simulink model "sim_velo_control_PD_a_b_cCompensate"  (R2020b)
settings: Solver=FixedStepAuto  StartTime=0.0  StopTime=120  FixedStep=0.01  RelTol=1e-3
libraries: pid_lib x1
settings Model: Creator=User  LastModifiedBy=tuna
settings ConfigComp: PLC_TargetIDE=codesys23

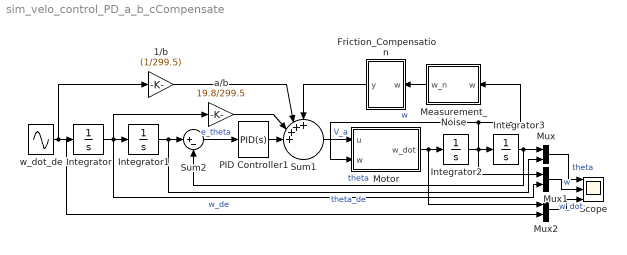
== system sim_velo_control_PD_a_b_cCompensate ==
  1/b : Gain  Gain=(1/299.5)
  Friction_Compensation : MATLAB Function  TreatAsAtomicUnit=on
  Integrator : Integrator  InitialCondition=15
  Integrator1 : Integrator
  Integrator2 : Integrator
  Integrator3 : Integrator
  Measurement_Noise : MATLAB Function  TreatAsAtomicUnit=on
  Motor : MATLAB Function  TreatAsAtomicUnit=on
  Mux : Mux  Inputs=2
  Mux1 : Mux  Inputs=2
  Mux2 : Mux  Inputs=2
  PID Controller1 : pid_lib/PID Controller  Controller=PID  Form=Parallel  TimeDomain=Continuous-time  UseExternalTs=off  SampleTime=-1  IntegratorMethod=Forward Euler  FilterMethod=Forward Euler  ControllerParametersSource=internal  P=3.8093  I=0  D=0.1596  UseFilter=on  N=100  TunerSelectOption=Transfer Function Based (PID Tuner App)  InitialConditionSource=internal  InitialConditionForIntegrator=0  InitialConditionForFilter=0  DifferentiatorICPrevScaledInput=0  ExternalReset=none  TrackingMode=off  Kt=1  LimitOutput=off  SatLimitsSource=internal  UpperSaturationLimit=inf  LowerSaturationLimit=-inf  LinearizeAsGain=on  AntiWindupMode=none  Kb=1  POutMin=[]  POutMax=[]  IOutMin=[]  IOutMax=[]  DOutMin=[]  DOutMax=[]  NOutMin=[]  NOutMax=[]  SumOutMin=[]  SumOutMax=[]  SaturationOutMin=[]  SaturationOutMax=[]  PParamMin=[]  PParamMax=[]  IParamMin=[]  IParamMax=[]  DParamMin=[]  DParamMax=[]  NParamMin=[]  NParamMax=[]  KbParamMin=[]  KbParamMax=[]  KtParamMin=[]  KtParamMax=[]  KbOutMin=[]  KbOutMax=[]  KtOutMin=[]  KtOutMax=[]  IntegratorOutMin=[]  IntegratorOutMax=[]  FilterOutMin=[]  FilterOutMax=[]  SumI1OutMin=[]  SumI1OutMax=[]  SumI2OutMin=[]  SumI2OutMax=[]  SumI3OutMin=[]  SumI3OutMax=[]  SumI4OutMin=[]  SumI4OutMax=[]  SumDOutMin=[]  SumDOutMax=[]  DifferentiatorOutMin=[]  DifferentiatorOutMax=[]  FilterDiffOutCoefMin=[]  FilterDiffOutCoefMax=[]  ReciprocalOutMin=[]  ReciprocalOutMax=[]  SumDenOutMin=[]  SumDenOutMax=[]  SumNumOutMin=[]  SumNumOutMax=[]  DivideOutMin=[]  DivideOutMax=[]  UdiffTsProdOutMin=[]  UdiffTsProdOutMax=[]  NTsProdOutMin=[]  NTsProdOutMax=[]  UintegralTsProdOutMin=[]  UintegralTsProdOutMax=[]  UngainTsProdOutMin=[]  UngainTsProdOutMax=[]  IntegratorContinuousStateAttributes=''  IntegratorStateMustResolveToSignalObject=off  IntegratorRTWStateStorageClass=Auto  FilterContinuousStateAttributes=''  FilterStateMustResolveToSignalObject=off  FilterRTWStateStorageClass=Auto  ParallelPVariant=InternalParameters  IdealPVariant=Disabled  IVariant=InternalParameters  DVariant=InternalParameters  IntegratorVariant=Continuous  SatVariant=Disabled  AWVariant=Passthrough  PCopyVariant=Disabled  TRVariant=Disabled  FdbkBlocksVariant=Forward  IdealPFdbkVariant=Disabled  SatFdbkVariant=Disabled  DerivativeFilterVariant=ContFilter  NVariant=InternalParameters  NCopyVariant=Disabled  FilterICVariant=InternalICsFilter  IntegratorICVariant=InternalICs  ExternalResetVariant=Disabled  TRSumVariant=Passthrough  SumFdbkVariant=Disabled  SumVariant=Sum_PID  TsampFilterVariant=InternalTs  TsampNgainVariant=Passthrough  TsampIntegralVariant=Passthrough  ExternalSaturationOutDataTypeStr=Inherit: Same as second input
  Scope : Scope  NumInputPorts=3
  Sum1 : Sum  Inputs=++++|||
  Sum2 : Sum  Inputs=|+-
  a/b : Gain  Gain=19.8/299.5
  w_dot_de : Sin  Amplitude=-22.5  Frequency=1.5  SampleTime=0
  wires:
  Sum2/1 -> PID Controller1/1  "e_theta"
  w_dot_de/1 -> 1/b/1, Mux2/2, Integrator/1
  Integrator3/1 -> Sum2/2, Mux/1  "theta"
  Sum1/1 -> Motor/1(u)  "V_a"
  Integrator1/1 -> Mux/2, Sum2/1  "theta_de"
  Motor/1(w_dot) -> Mux2/1, Integrator2/1
  Mux/1 -> Scope/1  "theta"
  Mux1/1 -> Scope/2  "w"
  Mux2/1 -> Scope/3  "w_dot"
  PID Controller1/1 -> Sum1/4
  Integrator/1 -> a/b/1, Mux1/2, Integrator1/1  "w_de"
  Integrator2/1 -> Motor/2(w), Measurement_Noise/1(w), Mux1/1, Integrator3/1  "w"
  Measurement_Noise/1(w_n) -> Friction_Compensation/1(w)
  a/b/1 -> Sum1/3
  1/b/1 -> Sum1/2
  Friction_Compensation/1(y) -> Sum1/1

== matlab function sim_velo_control_PD_a_b_cCompensate/Motor ==
  settings: updateMethod=DISCRETE
  data: u input; w_dot output; w input
function w_dot = fcn(u,w)
a= 20.0; %19.8;
b= 300.0; %299.5;
c= 10.0; %10.3;
w_dot = -a*w+b*u-c*sign(w);
w_dot = w_dot+ (0.01*randn(size(w_dot)))

== matlab function sim_velo_control_PD_a_b_cCompensate/Friction_Compensation ==
  data: w input; y output
function y = fcn(w)
c = 10.3;
b = 299.5;
y = (c/b) * sign(w);

== matlab function sim_velo_control_PD_a_b_cCompensate/Measurement_Noise ==
  settings: updateMethod=DISCRETE
  data: w input; w_n output
function w_n = fcn(w)
%#codegen

w_n = w + (0.01*randn(size(w)))
